simulink model "RC_Tiefpass_Wechselspannung_2016"  (R2016a)
settings: Solver=FixedStepAuto  SolverMode=SingleTasking  StartTime=0.0  StopTime=0.5  FixedStep=100e-6  RelTol=1e-3
undefined symbols (not defined in the file): C, d, R, T_PWM, ue_hat
settings Model: Creator=Gianluca  LastModifiedBy=Gianluca
settings DataIOCC: ReturnWorkspaceOutputs=on
settings DebuggingCC: UnconnectedInputMsg=none  UnconnectedOutputMsg=none  UnconnectedLineMsg=none  SFUnexpectedBacktrackingDiag=error  SFNoUnconditionalDefaultTransitionDiag=error
settings SFSimCC: SimUseLocalCustomCode=on
settings RTWCC: RTWUseLocalCustomCode=on
settings GRTTargetCC: TargetLangStandard=C99 (ISO)
settings ConfigComp: CovMetricSettings=dwe  CovSaveCumulativeToWorkspaceVar=off  CovSaveSingleToWorkspaceVar=off  CovExternalEMLEnable=on

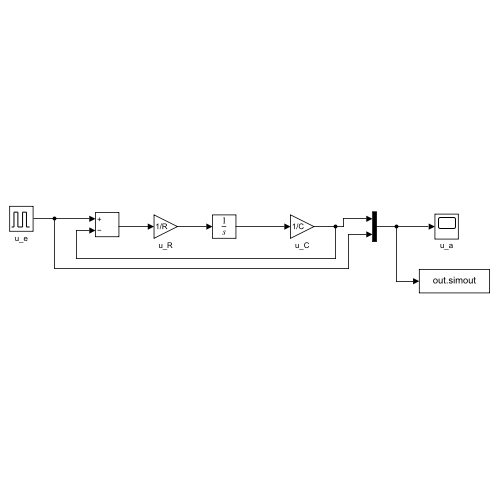
[thumbnail: Simulink's stored preview of the top-level diagram]
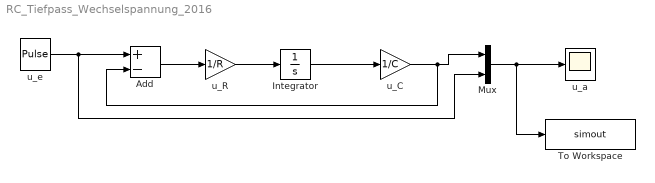
== system RC_Tiefpass_Wechselspannung_2016 ==
  Add : Sum  Inputs=+-
  Integrator : Integrator
  Mux : Mux  Inputs=2
  To Workspace : ToWorkspace  VariableName=simout  SaveFormat=Timeseries  SampleTime=-1
  u_C : Gain  Gain=1/C
  u_R : Gain  Gain=1/R
  u_a : Scope
  u_e : DiscretePulseGenerator  PulseType=Time based  Amplitude=ue_hat  Period=T_PWM  PulseWidth=d
  wires:
  u_e/1 -> Mux/2, Add/1
  Add/1 -> u_R/1
  Integrator/1 -> u_C/1
  u_R/1 -> Integrator/1
  Mux/1 -> To Workspace/1, u_a/1
  u_C/1 -> Add/2, Mux/1
